simulink model "BrakeJenkins"  (R2020b)
settings: Solver=ode1  StartTime=0.0  StopTime=inf  FixedStep=0.001  RelTol=1e-3
PreLoadFcn:
  | vehicle = 'Car'; if ~length(which('cmself')), cmenv; end
  | BrakeJenkins_bus
InitFcn:
  | vehicle = 'Car'; if ~length(which('cmself')), cmenv; end
  | BrakeJenkins_bus
Description:
  | CarMaker Plug-in Model Target
settings Model: Creator=giri.aigalikar  LastModifiedBy=giri.aigalikar
settings RTWCC: Description=CarMaker Plug-in Model Target  SystemTargetFile=CarMaker.tlc  TemplateMakefile=CarMaker_unix-win64.tmf
settings CodeAppCC: MaxIdLength=127
settings STFCustomTargetCC: TargetLangStandard=C99 (ISO)  ConcurrentExecutionCompliant=off  CombineOutputUpdateFcns=on  CodeInterfacePackaging=Reusable function  CPPClassGenCompliant=off  GRTInterface=off  GenerateAllocFcn=on  SystemTargetFile=CarMaker.tlc
settings GRTTargetCC: ParMdlRefBuildCompliant=off  CompOptLevelCompliant=off  ConcurrentExecutionCompliant=off  MatFileLogging=off  CodeInterfacePackaging=Reusable function  CPPClassGenCompliant=off  GenerateAllocFcn=on  UseToolchainInfoCompliant=off

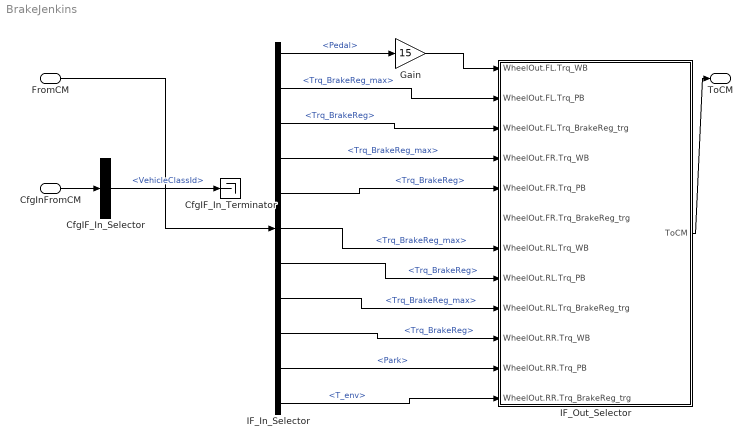
== system BrakeJenkins ==
  FromCM : Inport  OutDataTypeStr=Bus: cmBrakeIn
  CfgInFromCM : Inport  Port=2  OutDataTypeStr=Bus: cmBrakeCfgIn
  CfgIF_In_Selector : BusSelector  OutputSignals=VehicleClassId
  CfgIF_In_Terminator : Terminator
  Gain : Gain  Gain=15
  IF_In_Selector : BusSelector  OutputSignals=Pedal,WheelIn.FL.Trq_BrakeReg_max,WheelIn.FL.Trq_BrakeReg,WheelIn.FR.Trq_BrakeReg_max,WheelIn.FR.Trq_BrakeReg,WheelIn.RL.Trq_BrakeReg_max,WheelIn.RL.Trq_BrakeReg,WheelIn.RR.Trq_BrakeReg_max,WheelIn.RR.Trq_BrakeReg,Park,T_env
  IF_Out_Selector : Subsystem  mask(Signal Selection){}
      mask help: Signal Selection Block
      settings: OpenFcn=cmSignalSelect('SignalSelection_CB',gcb)
  ToCM : Outport  OutDataTypeStr=Bus: cmBrakeOut
  wires:
  FromCM/1 -> IF_In_Selector/1
  IF_Out_Selector/1(ToCM) -> ToCM/1
  CfgInFromCM/1 -> CfgIF_In_Selector/1
  CfgIF_In_Selector/1 -> CfgIF_In_Terminator/1  "<VehicleClassId>"
  IF_In_Selector/2 -> IF_Out_Selector/2(WheelOut.FL.Trq_PB)  "<Trq_BrakeReg_max>"
  IF_In_Selector/3 -> IF_Out_Selector/3(WheelOut.FL.Trq_BrakeReg_trg)  "<Trq_BrakeReg>"
  IF_In_Selector/4 -> IF_Out_Selector/4(WheelOut.FR.Trq_WB)  "<Trq_BrakeReg_max>"
  IF_In_Selector/5 -> IF_Out_Selector/5(WheelOut.FR.Trq_PB)  "<Trq_BrakeReg>"
  IF_In_Selector/6 -> IF_Out_Selector/7(WheelOut.RL.Trq_WB)  "<Trq_BrakeReg_max>"
  IF_In_Selector/7 -> IF_Out_Selector/8(WheelOut.RL.Trq_PB)  "<Trq_BrakeReg>"
  IF_In_Selector/8 -> IF_Out_Selector/9(WheelOut.RL.Trq_BrakeReg_trg)  "<Trq_BrakeReg_max>"
  IF_In_Selector/9 -> IF_Out_Selector/10(WheelOut.RR.Trq_WB)  "<Trq_BrakeReg>"
  IF_In_Selector/10 -> IF_Out_Selector/11(WheelOut.RR.Trq_PB)  "<Park>"
  IF_In_Selector/11 -> IF_Out_Selector/12(WheelOut.RR.Trq_BrakeReg_trg)  "<T_env>"
  IF_In_Selector/1 -> Gain/1  "<Pedal>"
  Gain/1 -> IF_Out_Selector/1(WheelOut.FL.Trq_WB)

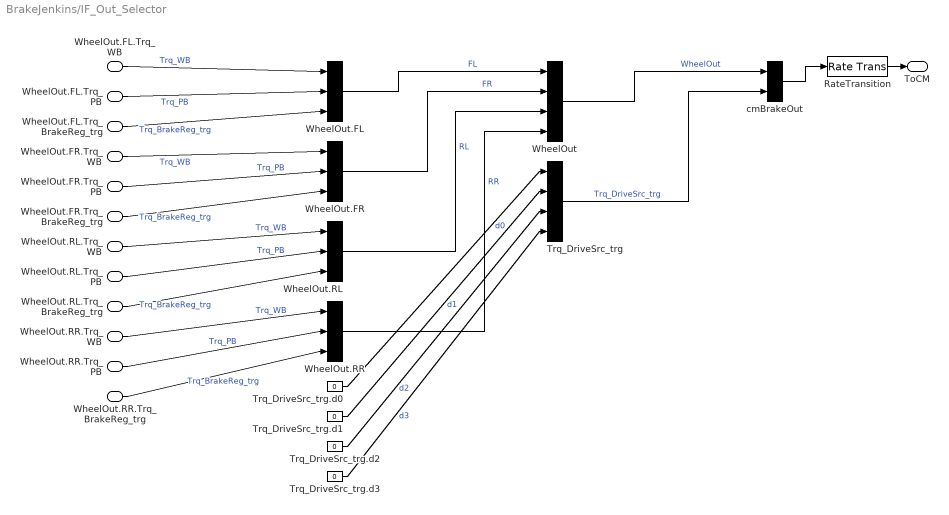
== system BrakeJenkins/IF_Out_Selector ==
  WheelOut.FL.Trq_WB : Inport
  WheelOut.FL.Trq_PB : Inport  Port=2
  WheelOut.FL.Trq_BrakeReg_trg : Inport  Port=3
  WheelOut.FR.Trq_WB : Inport  Port=4
  WheelOut.FR.Trq_PB : Inport  Port=5
  WheelOut.FR.Trq_BrakeReg_trg : Inport  Port=6
  WheelOut.RL.Trq_WB : Inport  Port=7
  WheelOut.RL.Trq_PB : Inport  Port=8
  WheelOut.RL.Trq_BrakeReg_trg : Inport  Port=9
  WheelOut.RR.Trq_WB : Inport  Port=10
  WheelOut.RR.Trq_PB : Inport  Port=11
  WheelOut.RR.Trq_BrakeReg_trg : Inport  Port=12
  RateTransition : RateTransition  OutPortSampleTime=str2num(get_param(bdroot,'FixedStep'))
  Trq_DriveSrc_trg : BusCreator  Inputs=4
  Trq_DriveSrc_trg.d{0..3} (4 alike) : Constant  Value=0
  WheelOut : BusCreator  Inputs=4
  WheelOut.FL : BusCreator  Inputs=3
  WheelOut.FR : BusCreator  Inputs=3
  WheelOut.RL : BusCreator  Inputs=3
  WheelOut.RR : BusCreator  Inputs=3
  cmBrakeOut : BusCreator  Inputs=2
  ToCM : Outport
  wires:
  RateTransition/1 -> ToCM/1
  cmBrakeOut/1 -> RateTransition/1
  WheelOut/1 -> cmBrakeOut/1  "WheelOut"
  WheelOut.FL/1 -> WheelOut/1  "FL"
  WheelOut.FR/1 -> WheelOut/2  "FR"
  WheelOut.RL/1 -> WheelOut/3  "RL"
  WheelOut.RR/1 -> WheelOut/4  "RR"
  Trq_DriveSrc_trg/1 -> cmBrakeOut/2  "Trq_DriveSrc_trg"
  WheelOut.FL.Trq_WB/1 -> WheelOut.FL/1  "Trq_WB"
  WheelOut.FL.Trq_PB/1 -> WheelOut.FL/2  "Trq_PB"
  WheelOut.FL.Trq_BrakeReg_trg/1 -> WheelOut.FL/3  "Trq_BrakeReg_trg"
  WheelOut.FR.Trq_WB/1 -> WheelOut.FR/1  "Trq_WB"
  WheelOut.FR.Trq_PB/1 -> WheelOut.FR/2  "Trq_PB"
  WheelOut.FR.Trq_BrakeReg_trg/1 -> WheelOut.FR/3  "Trq_BrakeReg_trg"
  WheelOut.RL.Trq_WB/1 -> WheelOut.RL/1  "Trq_WB"
  WheelOut.RL.Trq_PB/1 -> WheelOut.RL/2  "Trq_PB"
  WheelOut.RL.Trq_BrakeReg_trg/1 -> WheelOut.RL/3  "Trq_BrakeReg_trg"
  WheelOut.RR.Trq_WB/1 -> WheelOut.RR/1  "Trq_WB"
  WheelOut.RR.Trq_PB/1 -> WheelOut.RR/2  "Trq_PB"
  WheelOut.RR.Trq_BrakeReg_trg/1 -> WheelOut.RR/3  "Trq_BrakeReg_trg"
  Trq_DriveSrc_trg.d0/1 -> Trq_DriveSrc_trg/1  "d0"
  Trq_DriveSrc_trg.d1/1 -> Trq_DriveSrc_trg/2  "d1"
  Trq_DriveSrc_trg.d2/1 -> Trq_DriveSrc_trg/3  "d2"
  Trq_DriveSrc_trg.d3/1 -> Trq_DriveSrc_trg/4  "d3"
